simulink model "mhe_testing1"  (R2023b)
settings: Solver=VariableStepAuto  StartTime=0.0  StopTime=30  RelTol=1e-3
values from neighbouring files (symbols this model uses):
  Ts = 0.05    [NMPC_CSTR.m]
settings Model: Creator=akeebismail  LastModifiedBy=akeebismail

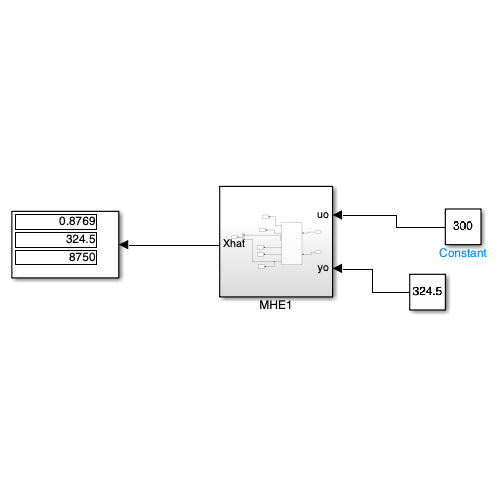
[thumbnail: Simulink's stored preview of the top-level diagram]
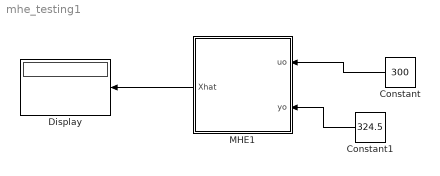
== system mhe_testing1 ==
  Constant : Constant  Value=300
  Constant1 : Constant  Value=324.5
  Display : Display
  MHE1 : Subsystem
  wires:
  Constant/1 -> MHE1/1(uo)
  Constant1/1 -> MHE1/2(yo)
  MHE1/1(Xhat) -> Display/1

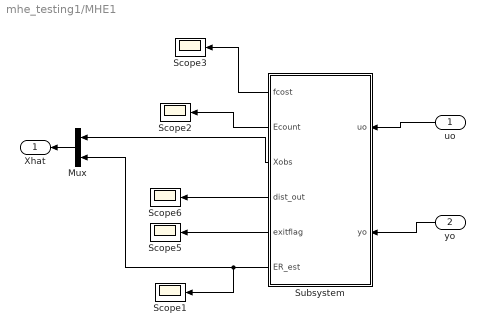
== system mhe_testing1/MHE1 ==
  uo : Inport
  yo : Inport  Port=2
  Mux : Mux  Inputs=2
  Scope{1..3,5..6} (5 alike) : Scope
  Subsystem : Subsystem
  Xhat : Outport
  wires:
  uo/1 -> Subsystem/1(uo)
  yo/1 -> Subsystem/2(yo)
  Subsystem/1(fcost) -> Scope3/1
  Subsystem/2(Ecount) -> Scope2/1
  Subsystem/6(ER_est) -> Mux/2, Scope1/1
  Subsystem/5(exitflag) -> Scope5/1
  Subsystem/4(dist_out) -> Scope6/1
  Mux/1 -> Xhat/1
  Subsystem/3(Xobs) -> Mux/1

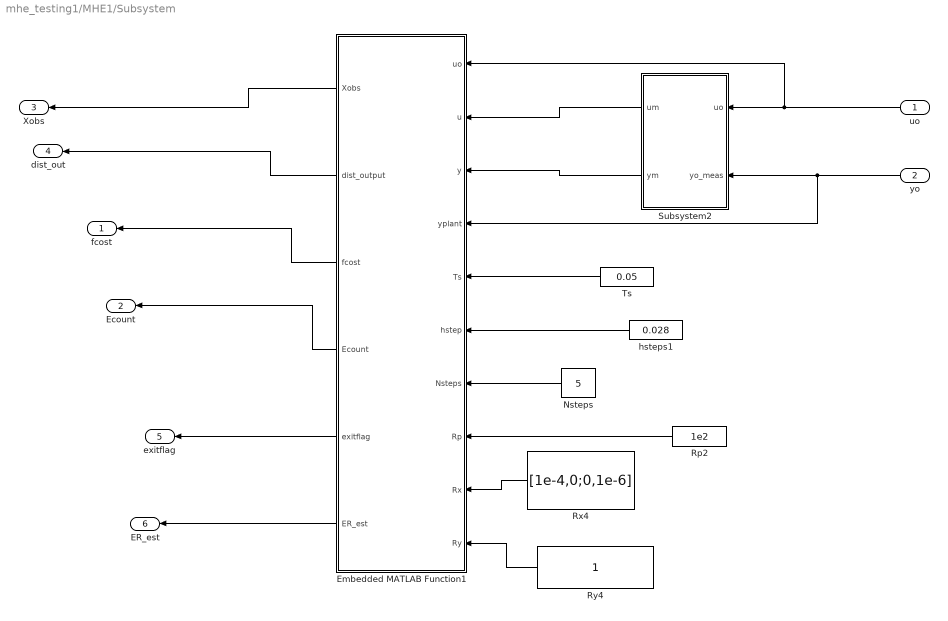
== system mhe_testing1/MHE1/Subsystem ==
  uo : Inport
  yo : Inport  Port=2
  Embedded MATLAB Function1 : MATLAB Function  TreatAsAtomicUnit=on
  Nsteps : Constant  Value=5
  Rp2 : Constant  Value=1e2
  Rx4 : Constant  Value=[1e-4,0;0,1e-6]
  Ry4 : Constant
  Subsystem2 : Subsystem
  Ts : Constant  Value=0.05
  hsteps1 : Constant  Value=0.028
  fcost : Outport  VectorParamsAs1DForOutWhenUnconnected=off
  Ecount : Outport  Port=2  VectorParamsAs1DForOutWhenUnconnected=off
  Xobs : Outport  Port=3  VectorParamsAs1DForOutWhenUnconnected=off
  dist_out : Outport  Port=4  VectorParamsAs1DForOutWhenUnconnected=off
  exitflag : Outport  Port=5  VectorParamsAs1DForOutWhenUnconnected=off
  ER_est : Outport  Port=6  VectorParamsAs1DForOutWhenUnconnected=off
  wires:
  Subsystem2/1(um) -> Embedded MATLAB Function1/2(u)
  Subsystem2/2(ym) -> Embedded MATLAB Function1/3(y)
  yo/1 -> Embedded MATLAB Function1/4(yplant), Subsystem2/2(yo_meas)
  uo/1 -> Embedded MATLAB Function1/1(uo), Subsystem2/1(uo)
  Nsteps/1 -> Embedded MATLAB Function1/7(Nsteps)
  hsteps1/1 -> Embedded MATLAB Function1/6(hstep)
  Embedded MATLAB Function1/3(fcost) -> fcost/1
  Embedded MATLAB Function1/4(Ecount) -> Ecount/1
  Rp2/1 -> Embedded MATLAB Function1/8(Rp)
  Rx4/1 -> Embedded MATLAB Function1/9(Rx)
  Ry4/1 -> Embedded MATLAB Function1/10(Ry)
  Embedded MATLAB Function1/1(Xobs) -> Xobs/1
  Embedded MATLAB Function1/2(dist_output) -> dist_out/1
  Embedded MATLAB Function1/5(exitflag) -> exitflag/1
  Embedded MATLAB Function1/6(ER_est) -> ER_est/1
  Ts/1 -> Embedded MATLAB Function1/5(Ts)

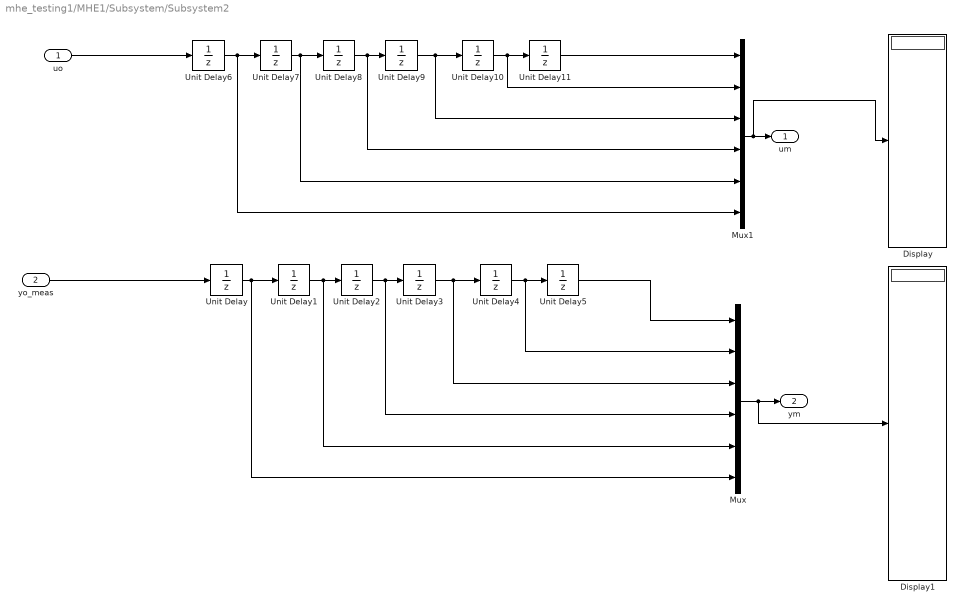
== system mhe_testing1/MHE1/Subsystem/Subsystem2 ==
  uo : Inport
  yo_meas : Inport  Port=2
  Display : Display
  Display1 : Display
  Mux : Mux  Inputs=6
  Mux1 : Mux  Inputs=6
  Unit Delay{,1..5} (6 alike) : UnitDelay  InitialCondition=324.5  SampleTime=Ts  HasFrameUpgradeWarning=on
  Unit Delay{6..11} (6 alike) : UnitDelay  InitialCondition=300  SampleTime=Ts  HasFrameUpgradeWarning=on
  um : Outport  VectorParamsAs1DForOutWhenUnconnected=off
  ym : Outport  Port=2  VectorParamsAs1DForOutWhenUnconnected=off
  wires:
  Unit Delay/1 -> Unit Delay1/1, Mux/6
  Unit Delay1/1 -> Unit Delay2/1, Mux/5
  Unit Delay2/1 -> Unit Delay3/1, Mux/4
  Unit Delay3/1 -> Unit Delay4/1, Mux/3
  Unit Delay4/1 -> Unit Delay5/1, Mux/2
  uo/1 -> Unit Delay6/1
  Unit Delay6/1 -> Mux1/6, Unit Delay7/1
  Unit Delay7/1 -> Mux1/5, Unit Delay8/1
  Unit Delay8/1 -> Mux1/4, Unit Delay9/1
  Unit Delay9/1 -> Mux1/3, Unit Delay10/1
  Unit Delay10/1 -> Unit Delay11/1, Mux1/2
  Mux/1 -> ym/1, Display1/1
  Mux1/1 -> um/1, Display/1
  Unit Delay11/1 -> Mux1/1
  Unit Delay5/1 -> Mux/1
  yo_meas/1 -> Unit Delay/1

== matlab function mhe_testing1/MHE1/Subsystem/Embedded MATLAB Function1 ==
  data: uo input; Xobs output size=[2,1]; dist_output output size=[1,1]; u input; y input; yplant input; Ts input; hstep input; Nsteps input; Rp input; fcost output size=[1,1]; Rx input; Ry input; Ecount output size=[1,1]; exitflag output size=[1,1]; ER_est output size=[1,1]
function [Xobs,dist_output,fcost,Ecount,exitflag,ER_est] =MHE(uo,u,y,yplant,Ts,hstep,Nsteps,Rp,Rx,Ry)

%#codegen
coder.extrinsic('MHE_compute','clear_var');

um=[u(1),u(2),u(3),u(4),u(5),u(6)] ;
 

ymeas=[y(1),y(2),y(3),y(4),y(5),y(6)] ;


    
   

% SAMPLING TIME FOR DISCRETIZATION
%hstep=1; %sampling time of 10 is with less interation while 5 is smoother but higher interaction
%Nsteps=1 ;% Nsteps=10 ; % Nsteps=20 ;


d_initial=[0.877;324.5;8750]   ;
%d_MIN_colvector =[0;0;100]  ;
d_MIN_colvector =[0.3;300;2000]  ;
d_MAX_colvector =[1.5;360;10000]  ;
%%%%%%%%%%%%%%%%%%%%%%%%%%%%%%%%%%%%%%%
%Initializing variables
fcost=inf  ;
Xobs=[0;0]  ;
%d_opt=[0;0]  ;
dist_output = [0]  ;
ER_est=[0]  ;
Ecount=0  ;
exitflag=2   ;

% [Xobs,dist_output,fcost,Ecount,exitflag]=MHE_compute(uo,um,ymeas,yplant...
%                                         ,hstep,Nsteps,Nmhe,Rp,Rx,Ry...
%                                         ,p_initial, p_MIN_colvector,p_MAX_colvector)
[Xobs,dist_output,ER_est,fcost,Ecount,exitflag]=MHE_compute(uo,um,ymeas...
                                        ,yplant,Ts,hstep,Nsteps,Rp,Rx,Ry...
                                        ,d_initial, d_MIN_colvector,d_MAX_colvector);
